simulink model "BE_Trotinette (1)"  (R2020a)
settings: Solver=VariableStepAuto  StartTime=0.0  StopTime=0.01  RelTol=1e-3
libraries: cstblocks x3, simulink x1
settings Model: Creator=menendez  LastModifiedBy=menendez

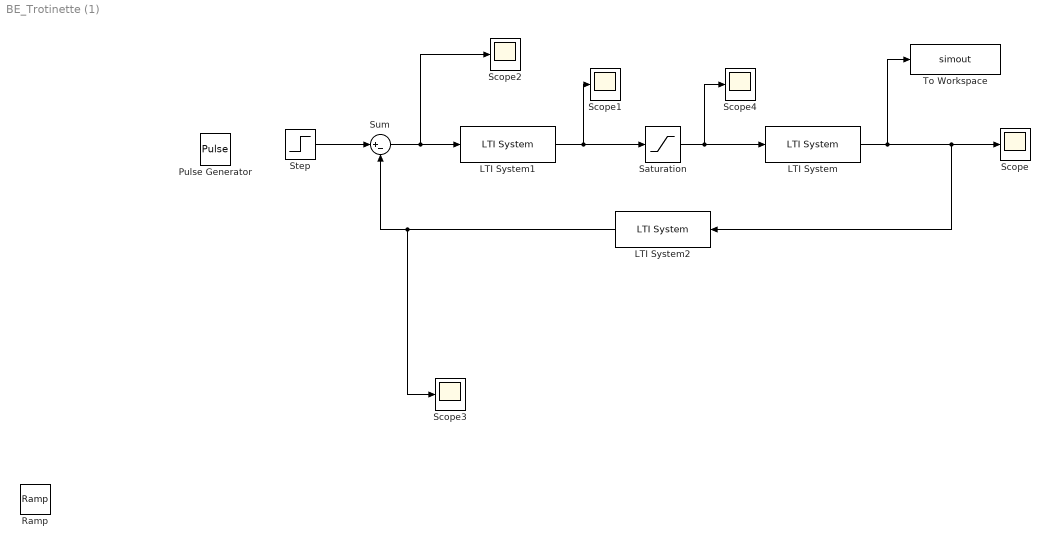
== system BE_Trotinette (1) ==
  LTI System : cstblocks/LTI System  sys=G  IC=[]
  LTI System1 : cstblocks/LTI System  sys=Cz1  IC=[]
  LTI System2 : cstblocks/LTI System  sys=F  IC=[]
  Pulse Generator : DiscretePulseGenerator  PulseType=Time based  Amplitude=0.1  Period=0.05  PulseWidth=50
  Ramp : simulink/Sources/Ramp  slope=0.1  start=0  InitialOutput=0
  Saturation : Saturate
  Scope{,1..4} (5 alike) : Scope
  Step : Step  Time=0.005  After=0.1  SampleTime=0
  Sum : Sum  Inputs=|+-
  To Workspace : ToWorkspace  VariableName=simout  SaveFormat=Timeseries  SampleTime=-1
  wires:
  Sum/1 -> Scope2/1, LTI System1/1
  LTI System/1 -> To Workspace/1, Scope/1, LTI System2/1
  LTI System1/1 -> Saturation/1, Scope1/1
  Saturation/1 -> Scope4/1, LTI System/1
  LTI System2/1 -> Scope3/1, Sum/2
  Step/1 -> Sum/1
